simulink model "T1_INT16_LREAL_mixed_scalar_200_aligned_RW_10ms"  (R2021b)
settings: Solver=VariableStepAuto  StartTime=0.0  StopTime=T_sim_end  RelTol=1e-3
model workspace (MAT data in the model file):
  ConnVar.ipAddress = '192.168.0.153'
  ConnVar.user = 'M1'
  ConnVar.pwd = [145 145 158 146 151 156 158 157]
  ConnVar.targetHandle = 0
values from neighbouring files (symbols this model uses):
  Ts_com = 0.1    [Script_individual_test_init.m]
undefined symbols (not defined in the file or in its folder): PLC_PRG, var1, var1_INT16_LREAL_scalar_bus_200_mixed_aligned_in, var1_INT16_LREAL_scalar_bus_200_mixed_aligned_out, var2, var3, var4
libraries: M1SWBlocks x2
settings Model: Creator=CHSE  LastModifiedBy=gione

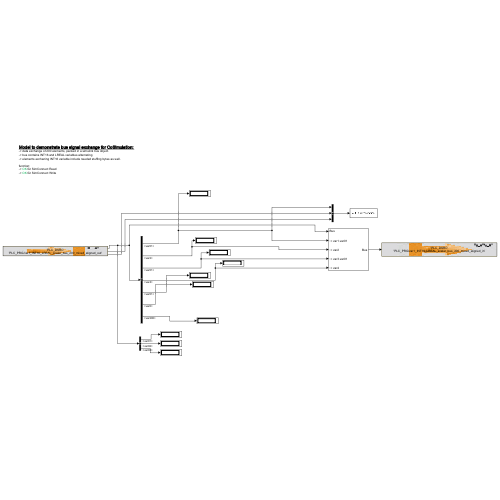
[thumbnail: Simulink's stored preview of the top-level diagram]
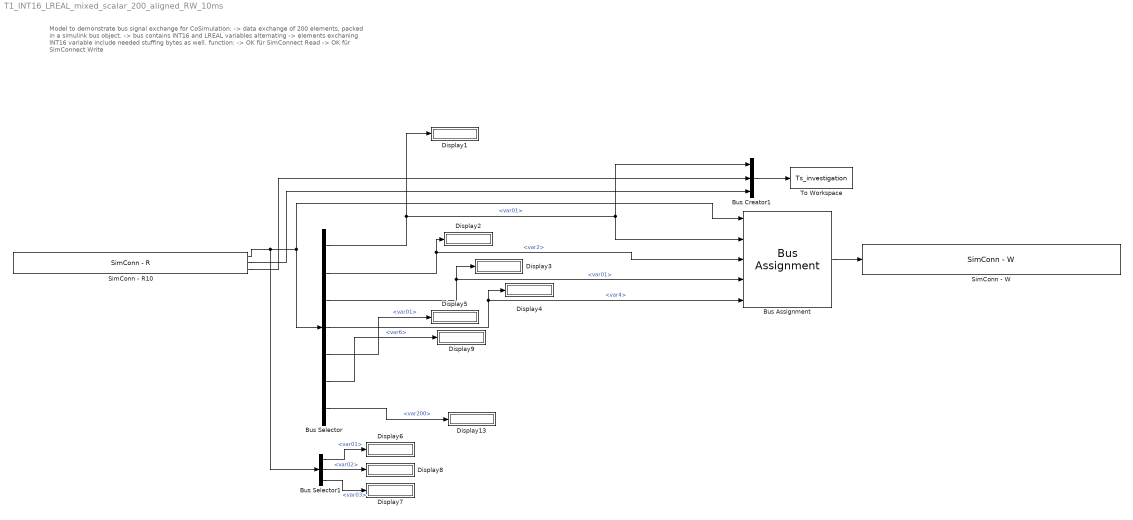
== system T1_INT16_LREAL_mixed_scalar_200_aligned_RW_10ms ==
  note: Model to demonstrate bus signal exchange for CoSimulation:
      | -> data exchange of 200 elements, packed in a simulink bus object.
      | -> bus contains INT16 and LREAL variables alternating
      | -> elements exchaning INT16 variable include needed stuffing bytes as well.
      |
      | function:
      | -> OK für SimConnect Read
      | -> OK für SimConnect Write
  Bus Assignment : BusAssignment  AssignedSignals=var1.var01,var2,var3.var01,var4
  Bus Creator1 : BusCreator  Inputs=3
  Bus Selector : BusSelector  OutputSignals=var1.var01,var2,var3.var01,var4,var5.var01,var6,var200
  Bus Selector1 : BusSelector  OutputSignals=var1.var01,var1.var02,var1.var03
  Display{1..9,13} (10 alike) : Display
  SimConn - R10 : M1SWBlocks/SimConn Blocks/SimConn - R  connVarName=ConnVar  InswModuleName='PLC_DSRC'  swModuleName=PLC_DSRC  InvarName='PLC_PRG/var1_INT16_LREAL_scalar_bus_200_mixed_aligned_out'  varName=PLC_PRG/var1_INT16_LREAL_scalar_bus_200_mixed_aligned_out  varDataType=Bus: Bus_exchange_INT16_LREAL_mixed_scalar_200_aligned  enRetOutput=on  enGetTrigger=off  getTrigger=rising  valDurLostConn=Zero  internalVal=0  DataDim=1  enSampTimMon=on  sampleTime=Ts_com
      settings: SourceProductName=Bachmann M1 Software
  SimConn - W : M1SWBlocks/SimConn Blocks/SimConn - W  connVarName=ConnVar  InswModuleName='PLC_DSRC'  swModuleName=PLC_DSRC  InvarName='PLC_PRG/var1_INT16_LREAL_scalar_bus_200_mixed_aligned_in'  varName=PLC_PRG/var1_INT16_LREAL_scalar_bus_200_mixed_aligned_in  varDataType=Bus: Bus_exchange_INT16_LREAL_mixed_scalar_200_aligned  enRetOutput=off  enGetTrigger=off  getTrigger=rising  enSampTimMon=off
      settings: SourceProductName=Bachmann M1 Software
  To Workspace : ToWorkspace  VariableName=Ts_investigation  SaveFormat=Timeseries  SampleTime=Ts_com
  wires:
  Bus Selector/2 -> Display2/1, Bus Assignment/3  "<var2>"
  Bus Selector/3 -> Display3/1, Bus Assignment/4  "<var01>"
  Bus Selector/4 -> Display4/1, Bus Assignment/5  "<var4>"
  Bus Creator1/1 -> To Workspace/1
  Bus Selector/1 -> Display1/1, Bus Assignment/2, Bus Creator1/1  "<var01>"
  SimConn - R10/2 -> Bus Creator1/3
  SimConn - R10/1 -> Bus Selector1/1, Bus Selector/1, Bus Assignment/1
  Bus Selector1/1 -> Display6/1  "<var01>"
  Bus Selector1/3 -> Display7/1  "<var03>"
  Bus Selector1/2 -> Display8/1  "<var02>"
  Bus Selector/5 -> Display5/1  "<var01>"
  Bus Selector/6 -> Display9/1  "<var6>"
  Bus Selector/7 -> Display13/1  "<var200>"
  SimConn - R10/3 -> Bus Creator1/2
  Bus Assignment/1 -> SimConn - W/1
